simulink model "test_system"  (R2016b)
settings: Solver=ode4  StartTime=0.0  StopTime=3500.0  FixedStep=0.1  RelTol=1e-3
libraries: simulink x5, fuzblock x2
settings Model: Creator=martin  LastModifiedBy=martin
settings OptimizationCC: DefaultParameterBehavior=Inlined  UseDivisionForNetSlopeComputation=on  UseFloatMulNetSlope=on  InlineInvariantSignals=on  PassReuseOutputArgsAs=Individual arguments  ZeroExternalMemoryAtStartup=off  ZeroInternalMemoryAtStartup=off  NoFixptDivByZeroProtection=on  EfficientFloat2IntCast=on  LifeSpan=1
settings DebuggingCC: ParameterTunabilityLossMsg=error
settings HardwareCC: ProdBitPerLong=64  ProdHWDeviceType=Intel->x86-64 (Linux 64)
settings RTWCC: SystemTargetFile=ert.tlc  TemplateMakefile=ert_default_tmf  Description=Embedded Coder  GenerateReport=on  IncludeHyperlinkInReport=on  LaunchReport=on  TargetLang=C++  GenerateTraceInfo=on  GenerateTraceReport=on  GenerateTraceReportSl=on  GenerateTraceReportSf=on  GenerateTraceReportEml=on
settings CodeAppCC: ForceParamTrailComments=on  IgnoreCustomStorageClasses=off  OperatorAnnotations=on  SimulinkDataObjDesc=on  SFDataObjDesc=on  MATLABFcnDesc=on  CustomSymbolStrGlobalVar=rt$N$M  CustomSymbolStrType=$N$M  CustomSymbolStrFcn=$N$M$F  CustomSymbolStrMacro=$N$M  InsertBlockDesc=on  MATLABSourceComments=on
settings ERTTargetCC: TargetLangStandard=C++03 (ISO)  GenerateSampleERTMain=on  CombineSignalStateStructs=on  SupportAbsoluteTime=off  MultiInstanceERTCode=on  CodeInterfacePackaging=C++ class  SupportComplex=off  SupportContinuousTime=on  InlinedParameterPlacement=NonHierarchical  RootIOFormat=Structure reference  ERTCustomFileTemplate=example_file_process.tlc  ERTFilePackagingFormat=CompactWithDataFile

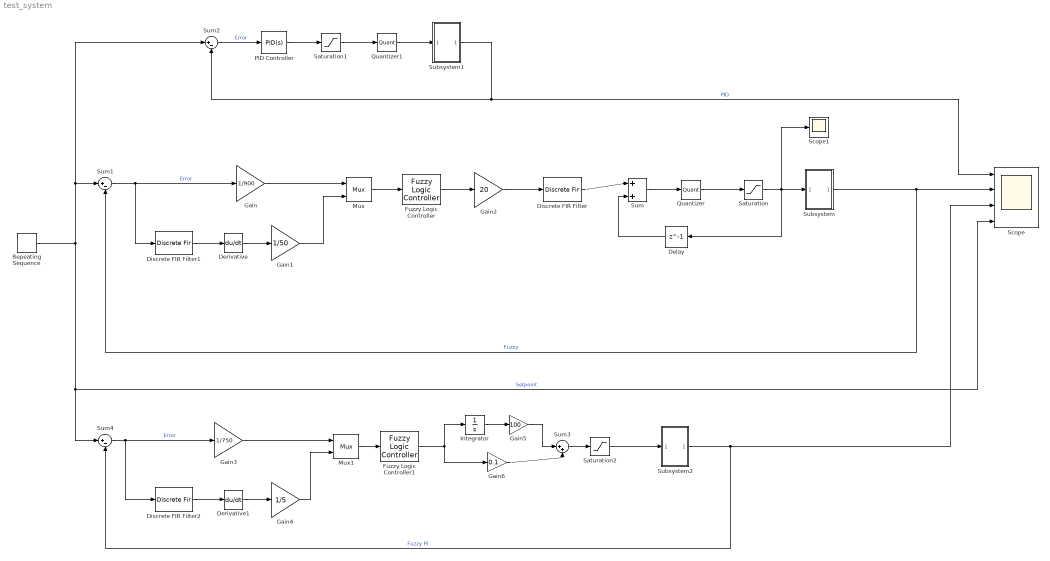
== system test_system ==
  Delay : Delay  DelayLength=1
  Derivative : Derivative
  Derivative1 : Derivative
  Discrete FIR Filter : DiscreteFir  Coefficients=[0.25 0.25 0.25 0.25]
  Discrete FIR Filter1 : DiscreteFir  Coefficients=[0.25 0.25 0.25 0.25]
  Discrete FIR Filter2 : DiscreteFir  Coefficients=[0.25 0.25 0.25 0.25]
  Fuzzy Logic Controller : fuzblock/Fuzzy Logic  Controller  fis='2x1.fis'
  Fuzzy Logic Controller1 : fuzblock/Fuzzy Logic  Controller  fis='2x1_pid.fis'
  Gain : Gain  Gain=1/900
  Gain1 : Gain  Gain=1/50
  Gain2 : Gain  Gain=20
  Gain3 : Gain  Gain=1/750
  Gain4 : Gain  Gain=1/5
  Gain5 : Gain  Gain=100
  Gain6 : Gain  Gain=0.1
  Integrator : Integrator
  Mux : Mux  Inputs=2
      settings: DisplayOption=signals
  Mux1 : Mux  Inputs=2
      settings: DisplayOption=signals
  PID Controller : simulink/Continuous/PID Controller  Controller=PID  TimeDomain=Continuous-time  SampleTime=-1  IntegratorMethod=Forward Euler  FilterMethod=Forward Euler  Form=Parallel  UseFilter=on  ControllerParametersSource=internal  P=4  I=0.001  D=0  N=100  InitialConditionSource=internal  InitialConditionForIntegrator=0  InitialConditionForFilter=0  ExternalReset=none  LimitOutput=off  UpperSaturationLimit=inf  LowerSaturationLimit=-inf  LinearizeAsGain=on  AntiWindupMode=none  Kb=1  TrackingMode=off  Kt=1  PParamMin=[]  PParamMax=[]  IParamMin=[]  IParamMax=[]  DParamMin=[]  DParamMax=[]  NParamMin=[]  NParamMax=[]  KbParamMin=[]  KbParamMax=[]  KtParamMin=[]  KtParamMax=[]  POutMin=[]  POutMax=[]  IOutMin=[]  IOutMax=[]  DOutMin=[]  DOutMax=[]  NOutMin=[]  NOutMax=[]  KbOutMin=[]  KbOutMax=[]  KtOutMin=[]  KtOutMax=[]  IntegratorOutMin=[]  IntegratorOutMax=[]  FilterOutMin=[]  FilterOutMax=[]  SumOutMin=[]  SumOutMax=[]  SumI1OutMin=[]  SumI1OutMax=[]  SumI2OutMin=[]  SumI2OutMax=[]  SumI3OutMin=[]  SumI3OutMax=[]  SumDOutMin=[]  SumDOutMax=[]  SaturationOutMin=[]  SaturationOutMax=[]  IntegratorContinuousStateAttributes=''  IntegratorStateMustResolveToSignalObject=off  IntegratorRTWStateStorageClass=Auto  FilterContinuousStateAttributes=''  FilterStateMustResolveToSignalObject=off  FilterRTWStateStorageClass=Auto  DifferentiatorICPrevScaledInput=0  DifferentiatorOutMin=[]  DifferentiatorOutMax=[]
  Quantizer : Quantizer  QuantizationInterval=1
  Quantizer1 : Quantizer  QuantizationInterval=1
  Repeating Sequence : simulink/Sources/Repeating Sequence  rep_seq_t=[0 499 500 3500]  rep_seq_y=[900 900 1200 1200]
  Saturation : Saturate  UpperLimit=100  LowerLimit=0
  Saturation1 : Saturate  UpperLimit=100  LowerLimit=0
  Saturation2 : Saturate  UpperLimit=100  LowerLimit=0
  Scope : Scope  NumInputPorts=4
  Scope1 : Scope
  Subsystem : Subsystem
  Subsystem1 : Subsystem
  Subsystem2 : Subsystem
  Sum : Sum  Inputs=|++
  Sum1 : Sum  Inputs=|+-
  Sum2 : Sum  Inputs=|+-
  Sum3 : Sum  Inputs=|++
  Sum4 : Sum  Inputs=|+-
  wires:
  Fuzzy Logic Controller/1 -> Gain2/1
  Subsystem/1(Out1) -> Sum1/2, Scope/2  "Fuzzy"
  Mux/1 -> Fuzzy Logic Controller/1
  Derivative/1 -> Gain1/1
  Sum1/1 -> Gain/1, Discrete FIR Filter1/1  "Error"
  Saturation1/1 -> Quantizer1/1
  Sum2/1 -> PID Controller/1  "Error"
  PID Controller/1 -> Saturation1/1
  Gain/1 -> Mux/1
  Gain1/1 -> Mux/2
  Subsystem1/1(Out1) -> Scope/1, Sum2/2  "PID"
  Saturation/1 -> Scope1/1, Delay/1, Subsystem/1(In1)
  Delay/1 -> Sum/2
  Sum/1 -> Quantizer/1
  Repeating Sequence/1 -> Scope/4, Sum4/1, Sum1/1, Sum2/1  "Setpoint"
  Subsystem2/1(Out1) -> Sum4/2, Scope/3  "Fuzzy PI"
  Mux1/1 -> Fuzzy Logic Controller1/1
  Derivative1/1 -> Gain4/1
  Sum4/1 -> Gain3/1, Discrete FIR Filter2/1  "Error"
  Gain3/1 -> Mux1/1
  Gain4/1 -> Mux1/2
  Saturation2/1 -> Subsystem2/1(In1)
  Fuzzy Logic Controller1/1 -> Gain6/1, Integrator/1
  Integrator/1 -> Gain5/1
  Gain5/1 -> Sum3/1
  Sum3/1 -> Saturation2/1
  Gain6/1 -> Sum3/2
  Gain2/1 -> Discrete FIR Filter/1
  Discrete FIR Filter/1 -> Sum/1
  Discrete FIR Filter1/1 -> Derivative/1
  Discrete FIR Filter2/1 -> Derivative1/1
  Quantizer/1 -> Saturation/1
  Quantizer1/1 -> Subsystem1/1(In1)

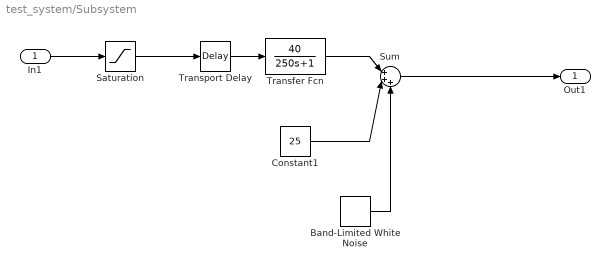
== system test_system/Subsystem ==
  In1 : Inport  OutMin=[0]  OutMax=[100]
  Band-Limited White Noise : simulink/Sources/Band-Limited White Noise  Cov=[0.1]  Ts=1  seed=[23341]
  Constant1 : Constant  Value=25
  Saturation : Saturate  UpperLimit=100  LowerLimit=0
  Sum : Sum  Inputs=|+++
  Transfer Fcn : TransferFcn  Numerator=[40]  Denominator=[250 1]
  Transport Delay : TransportDelay
  Out1 : Outport
  wires:
  Transfer Fcn/1 -> Sum/1
  Constant1/1 -> Sum/2
  Sum/1 -> Out1/1
  Transport Delay/1 -> Transfer Fcn/1
  In1/1 -> Saturation/1
  Saturation/1 -> Transport Delay/1
  Band-Limited White Noise/1 -> Sum/3

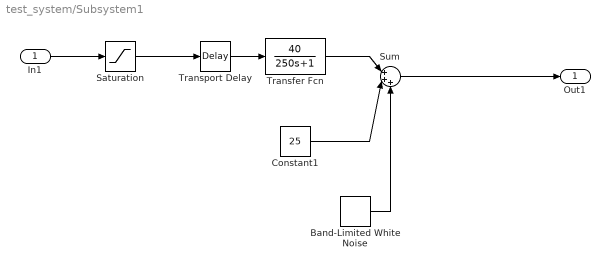
== system test_system/Subsystem1 ==
  In1 : Inport  OutMin=[0]  OutMax=[100]
  Band-Limited White Noise : simulink/Sources/Band-Limited White Noise  Cov=[0.1]  Ts=1  seed=[23341]
  Constant1 : Constant  Value=25
  Saturation : Saturate  UpperLimit=100  LowerLimit=0
  Sum : Sum  Inputs=|+++
  Transfer Fcn : TransferFcn  Numerator=[40]  Denominator=[250 1]
  Transport Delay : TransportDelay
  Out1 : Outport
  wires:
  Transfer Fcn/1 -> Sum/1
  Constant1/1 -> Sum/2
  Sum/1 -> Out1/1
  Transport Delay/1 -> Transfer Fcn/1
  In1/1 -> Saturation/1
  Saturation/1 -> Transport Delay/1
  Band-Limited White Noise/1 -> Sum/3

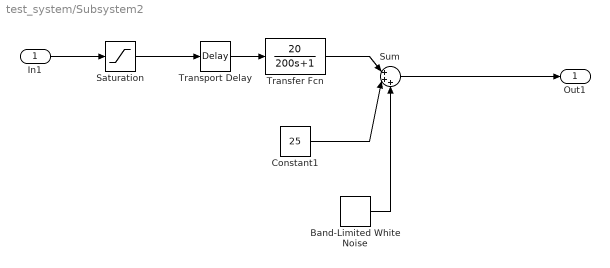
== system test_system/Subsystem2 ==
  In1 : Inport  OutMin=[0]  OutMax=[100]
  Band-Limited White Noise : simulink/Sources/Band-Limited White Noise  Cov=[0.1]  Ts=0.1  seed=[23341]
  Constant1 : Constant  Value=25
  Saturation : Saturate  UpperLimit=100  LowerLimit=0
  Sum : Sum  Inputs=|+++
  Transfer Fcn : TransferFcn  Numerator=[20]  Denominator=[200 1]
  Transport Delay : TransportDelay
  Out1 : Outport
  wires:
  Transfer Fcn/1 -> Sum/1
  Constant1/1 -> Sum/2
  Sum/1 -> Out1/1
  Transport Delay/1 -> Transfer Fcn/1
  In1/1 -> Saturation/1
  Saturation/1 -> Transport Delay/1
  Band-Limited White Noise/1 -> Sum/3
